simulink model "ejercicio_PI"  (R2025b)
settings: Solver=VariableStepAuto  StartTime=0.0  StopTime=10.0  RelTol=1e-3
undefined symbols (not defined in the file): K_de, K_du, K_e
libraries: fuzblock x1
settings Model: Creator=chenfu  LastModifiedBy=chenfu

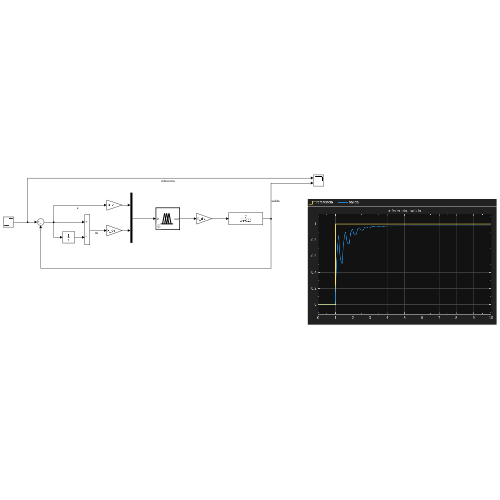
[thumbnail: Simulink's stored preview of the top-level diagram]
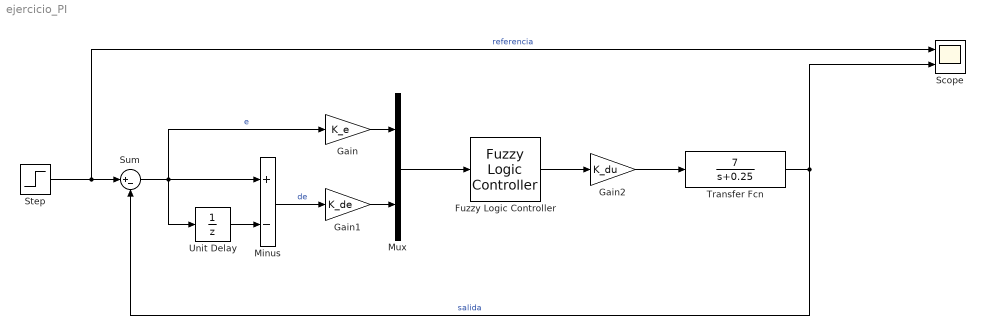
== system ejercicio_PI ==
  Fuzzy Logic Controller : fuzblock/Fuzzy Logic  Controller  FIS=fis  OutputSampleNumber=101  DataType=double  UseLookupTable=off  NumBreakpoints=10  FuzzifiedInputs=off  RuleFiringStrengths=off  RuleOutputs=off  AggregatedOutputs=off  SimulateUsing=Interpreted execution  OutOfRangeInputValueMessage=warning  NoRuleFiredMessage=warning  EmptyOutputFuzzySetMessage=warning
  Gain : Gain  Gain=K_e
  Gain1 : Gain  Gain=K_de
  Gain2 : Gain  Gain=K_du
  Minus : Sum  Inputs=+-
  Mux : Mux  Inputs=2
  Scope : Scope  NumInputPorts=2
      settings: ActiveDisplayYMinimum=-0.12500000000000003  ActiveDisplayYMaximum=1.125
  Step : Step  SampleTime=0
  Sum : Sum  Inputs=|+-
  Transfer Fcn : TransferFcn  Numerator=[7]  Denominator=[1 0.25]
  Unit Delay : UnitDelay  SampleTime=-1  HasFrameUpgradeWarning=on
  wires:
  Unit Delay/1 -> Minus/2
  Sum/1 -> Gain/1, Unit Delay/1, Minus/1  "e"
  Minus/1 -> Gain1/1  "de"
  Mux/1 -> Fuzzy Logic Controller/1
  Gain/1 -> Mux/1
  Gain1/1 -> Mux/2
  Fuzzy Logic Controller/1 -> Gain2/1
  Gain2/1 -> Transfer Fcn/1
  Step/1 -> Scope/1, Sum/1  "referencia"
  Transfer Fcn/1 -> Scope/2, Sum/2  "salida"
